simulink model "unicycle_lateral"  (R2019b)
settings: Solver=VariableStepAuto  StartTime=0.0  StopTime=20  RelTol=1e-3
values from neighbouring files (symbols this model uses):
  A = [0 1 0 0; 68747/250 0 -29463/250 0; 0 0 0 1;-19642/125 0 9821/125 0]    [test_2.m]    (also in test_3.m = [0 1 0 0; 35856471/2703500 0 -2857911/1081400 0; 0 0 0 1;-98; test_4.m = subs(jacobian(x1, x),[te,te1,a,a1,OA,AB,mB,g],x_equi); test_5.m = [0 1 0 0; 9821/750 0 -9821/2250 0; 0 0 0 1;0 0 9821/375 0]; unicycle.m = [0 1 0 0; 0 0 0 0; 0 0 0 1;0 0 5588149/150160 0])
  B = [0; -16/15; 0; 16/15]    [test_2.m]    (also in test_3.m = [0; -2250/5407; 0; 6925/5407]; test_4.m = subs(jacobian(x1, sym('M')),[te,te1,a,a1,OA,AB,mB,g],x_equi); test_5.m = [0;  -8/15; 0; 8/5]; unicycle.m = [0;  6250/17; 0; -12500/1877])
  K = place(A,B,eigs)    [test_2.m]    (also in test_3.m; test_4.m; unicycle.m = acker(A,B,eigs); unicycle_fro.m = place(A,B,eigs1))
libraries: simulink x1
settings Model: Creator=DooDooDude  LastModifiedBy=DooDooDude

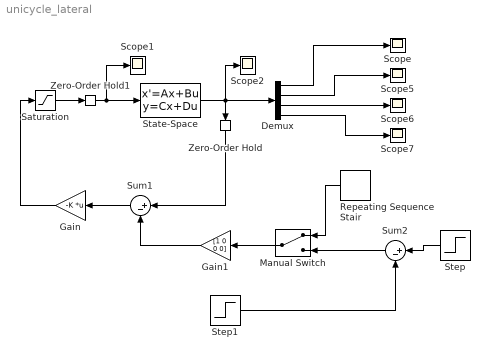
== system unicycle_lateral ==
  Demux : Demux
  Gain : Gain  Gain=-K  Multiplication=Matrix(K*u)
  Gain1 : Gain  Gain=[1 0 0 0]
  Manual Switch : ManualSwitch
  Repeating Sequence Stair : simulink/Sources/Repeating Sequence Stair  OutValues=[1 2 3 4 5 6 7 8 9 10 9 8 7 6 5 4 3 2 1 0].'  tsamp=0.5  OutMin=[]  OutMax=[]  OutDataTypeStr=double  OutputDataTypeScalingMode=double  OutDataType=fixdt(0,8)  ConRadixGroup=Best Precision: Vector-wise  OutScaling=2^-12
  Saturation : Saturate  UpperLimit=2  LowerLimit=-2
  Scope{,1..2,5..7} (6 alike) : Scope
  State-Space : StateSpace  A=A  B=B  C=eye(4)  D=[0; 0; 0; 0]  InitialCondition=[0; 0; 0; 0]
  Step : Step  SampleTime=0
  Step1 : Step  Time=2  SampleTime=0
  Sum1 : Sum  Inputs=|+-  InputSameDT=on
  Sum2 : Sum  Inputs=|+-  InputSameDT=on
  Zero-Order Hold : ZeroOrderHold  SampleTime=0.005
  Zero-Order Hold1 : ZeroOrderHold  SampleTime=0.005
  wires:
  Zero-Order Hold1/1 -> Scope1/1, State-Space/1
  Saturation/1 -> Zero-Order Hold1/1
  Gain/1 -> Saturation/1
  Zero-Order Hold/1 -> Sum1/1
  State-Space/1 -> Scope2/1, Demux/1, Zero-Order Hold/1
  Demux/1 -> Scope/1
  Demux/2 -> Scope5/1
  Demux/3 -> Scope6/1
  Demux/4 -> Scope7/1
  Sum1/1 -> Gain/1
  Gain1/1 -> Sum1/2
  Sum2/1 -> Manual Switch/2
  Step/1 -> Sum2/1
  Step1/1 -> Sum2/2
  Manual Switch/1 -> Gain1/1
  Repeating Sequence Stair/1 -> Manual Switch/1
